simulink model "MIL4L3_SW6_V1_20220211"  (R2018b)
settings: Solver=FixedStepAuto  StartTime=0.0  StopTime=inf  FixedStep=0.001  RelTol=1e-3
PreLoadFcn:
  | A0_MILtest;
undefined symbols (not defined in the file or in its folder): Clb_ICADirect_LaneDisp_StateFive, Clb_ICADirect_LaneDisp_StateFour, Clb_ICADirect_LaneDisp_StateOne, Clb_ICADirect_LaneDisp_StateThree, Clb_ICADirect_LaneDisp_StateTwo, Clb_ICADirect_LaneDisp_StateZero, Clb_ICADirect_LaneDispSW, Clb_ICADirect_TrnLghtsCom_Switch, Clb_ICADirect_TrnLghtsCom_Value, Clb_ICADirect_TrnLghtsCrtl_Inhb, IMAP_Clb_ACU_Driver_Belt, IMAP_Clb_ACU_Driver_Belt_Over, IMAP_Clb_ACU_Passenger_Belt, IMAP_Clb_ACU_Passenger_Belt_Over, IMAP_Clb_ACU_RearLeft_Belt, IMAP_Clb_ACU_RearLeft_Belt_Over, IMAP_Clb_ACU_RearMiddle_Belt, IMAP_Clb_ACU_RearMiddle_Belt_Over, IMAP_Clb_ACU_RearRight_Belt, IMAP_Clb_ACU_RearRight_Belt_Over, IMAP_Clb_AEB_Switch, IMAP_Clb_AEB_Switch_Over, IMAP_Clb_ALC_TLC_Mode, IMAP_Clb_ALC_TLC_Mode_Over, IMAP_Clb_BCM_Battery_Voltage, IMAP_Clb_BCM_Battery_Voltage_Over, IMAP_Clb_BCM_BrakeLamp_State, IMAP_Clb_BCM_BrakeLamp_State_Over, IMAP_Clb_BCM_CHMSL_Status, IMAP_Clb_BCM_CHMSL_Status_Over, IMAP_Clb_BCM_Door_Lock_State, IMAP_Clb_BCM_Door_Lock_State_Over, IMAP_Clb_BCM_FrontWiper_State, IMAP_Clb_BCM_FrontWiper_State_Over, IMAP_Clb_BCM_FrontWiper_Switch, IMAP_Clb_BCM_FrontWiper_Switch_Over, IMAP_Clb_BCM_HazardLamp, IMAP_Clb_BCM_HazardLamp_Over, IMAP_Clb_BCM_HazardLamp_Switch, IMAP_Clb_BCM_HazardLamp_Switch_Over, IMAP_Clb_BCM_HighBeam_State, IMAP_Clb_BCM_HighBeam_State_Over, IMAP_Clb_BCM_Ignition_State, IMAP_Clb_BCM_Ignition_State_Over, IMAP_Clb_BCM_IHBC_Enabled, IMAP_Clb_BCM_IHBC_Enabled_Over, IMAP_Clb_BCM_Left_Light, IMAP_Clb_BCM_Left_Light_Over, IMAP_Clb_BCM_LeftTurn_Switch, IMAP_Clb_BCM_LeftTurn_Switch_Over, IMAP_Clb_BCM_LF_Door_State, IMAP_Clb_BCM_LF_Door_State_Over, IMAP_Clb_BCM_LowBeam_State, IMAP_Clb_BCM_LowBeam_State_Over, IMAP_Clb_BCM_LR_Door_State, IMAP_Clb_BCM_LR_Door_State_Over, IMAP_Clb_BCM_RF_Door_State, IMAP_Clb_BCM_RF_Door_State_Over, IMAP_Clb_BCM_Right_Light, IMAP_Clb_BCM_Right_Light_Over ... (+547)
libraries: CarMaker4SL x2153, simulink x292, dspstat3 x3, canmsglib x2, simulink_extras x1
(part 39 of 52)

== system MIL4L3_SW6_V1_20220211/CarMaker/VehicleControl/Function/LKA/LKAS1/LL/LLOn/LKA Input Processing (LKAInP)/Previewed Heading Angle Calculation (PrHdAg) ==
  PrHdAg_bsInInfoSyn : Inport
  PrHdAg_bsLLClb : Inport  Port=2
  PrHdAg_bsTTLCInfo : Inport  Port=3
  Add1 : Sum  AccumDataTypeStr=single
  Add2 : Sum  AccumDataTypeStr=single
  Bus Creator1 : BusCreator  Inputs=8
  Bus Selector2 : BusSelector  OutputSignals=bsLaneInfo.bsL0Info,bsVehMovInfo.ESC_VehSpd,bsLaneInfo.bsR0Info
  Bus Selector3 : BusSelector  OutputSignals=bsLKAClb.LL_HdAgPrvwT_C
  Bus Selector4 : BusSelector  OutputSignals=LFTTTLC,RGTTTLC
  Compare To Constant : simulink/Logic and Bit Operations/Compare To Constant  relop=<=  const=2  OutDataTypeStr=boolean
  Compare To Constant1 : simulink/Logic and Bit Operations/Compare To Constant  relop=<=  const=2  OutDataTypeStr=boolean
  Gain1 : Gain  Gain=0.5
  Gain2 : Gain  Gain=0.5
  Perdicted Heading Angle from Right Lane Line (PrdcHdAgRgt)1 : Subsystem
  Perdicted Heading Angle from Right Lane Line (PrvwTTLCHdAgLftTTLCRgt) : Subsystem
  Perdicted Heading Angle from Right Lane Line (PrvwTTLCHdAgRgtTTLCRgt) : Subsystem
  Predicted Heading Angle from Left Lane Line (PrdcHdAgtLft)1 : Subsystem
  Predicted Heading Angle from Left Lane Line (PrdcHdAgtLftTTLCLft) : Subsystem
  Predicted Heading Angle from Left Lane Line (PrvwTTLCHdAgRgtTTLCLft) : Subsystem
  Saturation : Saturate  UpperLimit=2  LowerLimit=0.5
      settings: AttributesFormatString="Min = %<LowerLimit>  Max = %<UpperLimit>"
  Saturation1 : Saturate  UpperLimit=2  LowerLimit=0.5
      settings: AttributesFormatString="Min = %<LowerLimit>  Max = %<UpperLimit>"
  Switch : Switch  Criteria=u2 > Threshold
  Switch1 : Switch  Criteria=u2 > Threshold
  Z Calculation (ZCalc) : Subsystem
  Z Calculation (ZCalc)1 : Subsystem
  PrHdAg_bsPrHdAgInfo : Outport
  wires:
  PrHdAg_bsInInfoSyn/1 -> Bus Selector2/1
  Bus Selector2/3 -> Perdicted Heading Angle from Right Lane Line (PrvwTTLCHdAgRgtTTLCRgt)/2(PrdcHdAgRgt_bsR0Info), Perdicted Heading Angle from Right Lane Line (PrdcHdAgRgt)1/2(PrdcHdAgRgt_bsR0Info), Perdicted Heading Angle from Right Lane Line (PrvwTTLCHdAgLftTTLCRgt)/2(PrdcHdAgRgt_bsR0Info)  "<bsR0Info>"
  Z Calculation (ZCalc)/1(ZCalc_lPrvwDstZ) -> Perdicted Heading Angle from Right Lane Line (PrvwTTLCHdAgLftTTLCRgt)/1(PrdcHdAgRgt_lPrvwDstZ), Predicted Heading Angle from Left Lane Line (PrdcHdAgtLftTTLCLft)/2(PrdcHdAgtLft_lPrvwDstZ), Bus Creator1/6, Add1/1  "lPrvwZLft"
  Bus Selector4/1 -> Switch/1, Compare To Constant/1  "<LFTTTLC>"
  Bus Selector2/1 -> Predicted Heading Angle from Left Lane Line (PrvwTTLCHdAgRgtTTLCLft)/1(PrdcHdAgtLft_bsL0Info), Predicted Heading Angle from Left Lane Line (PrdcHdAgtLft)1/1(PrdcHdAgtLft_bsL0Info), Predicted Heading Angle from Left Lane Line (PrdcHdAgtLftTTLCLft)/1(PrdcHdAgtLft_bsL0Info)  "<bsL0Info>"
  Saturation/1 -> Z Calculation (ZCalc)/2(ZCalc_tiHdAgPrvwT_C)
  PrHdAg_bsTTLCInfo/1 -> Bus Selector4/1
  Bus Creator1/1 -> PrHdAg_bsPrHdAgInfo/1
  Bus Selector4/2 -> Switch1/1, Compare To Constant1/1  "<RGTTTLC>"
  Predicted Heading Angle from Left Lane Line (PrdcHdAgtLftTTLCLft)/1(PrdcHdAgtLft_phiPrdcHdAgLft) -> Bus Creator1/1  "phiPrvwTTLCHdAgLftTTLCLft"
  Perdicted Heading Angle from Right Lane Line (PrvwTTLCHdAgRgtTTLCRgt)/1(PrdcHdAgRgt_phiPrdcHdAgRgt) -> Bus Creator1/4  "phiPrvwTTLCHdAgRgtTTLCRgt"
  Bus Selector2/2 -> Z Calculation (ZCalc)1/1(ZCalc_vVehSpd), Z Calculation (ZCalc)/1(ZCalc_vVehSpd)  "<ESC_VehSpd>"
  Add2/1 -> Gain2/1
  Gain2/1 -> Bus Creator1/5  "phiPrvwHdAgMean"
  PrHdAg_bsLLClb/1 -> Bus Selector3/1
  Compare To Constant/1 -> Switch/2
  Switch/1 -> Saturation/1
  Switch1/1 -> Saturation1/1
  Bus Selector3/1 -> Switch/3, Switch1/3  "<LL_HdAgPrvwT_C>"
  Saturation1/1 -> Z Calculation (ZCalc)1/2(ZCalc_tiHdAgPrvwT_C)
  Z Calculation (ZCalc)1/1(ZCalc_lPrvwDstZ) -> Bus Creator1/7, Perdicted Heading Angle from Right Lane Line (PrvwTTLCHdAgRgtTTLCRgt)/1(PrdcHdAgRgt_lPrvwDstZ), Predicted Heading Angle from Left Lane Line (PrvwTTLCHdAgRgtTTLCLft)/2(PrdcHdAgtLft_lPrvwDstZ), Add1/2  "lPrvwZRgt"
  Compare To Constant1/1 -> Switch1/2
  Add1/1 -> Gain1/1
  Gain1/1 -> Predicted Heading Angle from Left Lane Line (PrdcHdAgtLft)1/2(PrdcHdAgtLft_lPrvwDstZ), Perdicted Heading Angle from Right Lane Line (PrdcHdAgRgt)1/1(PrdcHdAgRgt_lPrvwDstZ), Bus Creator1/8  "PrvwZMean"
  Predicted Heading Angle from Left Lane Line (PrdcHdAgtLft)1/1(PrdcHdAgtLft_phiPrdcHdAgLft) -> Add2/1  "phiPrvwTTLCHdAgLft"
  Perdicted Heading Angle from Right Lane Line (PrdcHdAgRgt)1/1(PrdcHdAgRgt_phiPrdcHdAgRgt) -> Add2/2  "phiPrvwTTLCHdAgRgt"
  Predicted Heading Angle from Left Lane Line (PrvwTTLCHdAgRgtTTLCLft)/1(PrdcHdAgtLft_phiPrdcHdAgLft) -> Bus Creator1/2  "phiPrvwTTLCHdAgRgtTTLCLft"
  Perdicted Heading Angle from Right Lane Line (PrvwTTLCHdAgLftTTLCRgt)/1(PrdcHdAgRgt_phiPrdcHdAgRgt) -> Bus Creator1/3  "phiPrvwTTLCHdAgLftTTLCRgt"

== system MIL4L3_SW6_V1_20220211/CarMaker/VehicleControl/Function/LKA/LKAS1/LL/LLOn/LKA Input Processing (LKAInP)/Steering Wheel Position Calculation (SWAPosCal) ==
  SWAPosCal_bsInInfoSyn : Inport
  SWAPosCal_bsLLClb : Inport  Port=2
  Bus Selector : BusSelector  OutputSignals=bsLaneInfo.bsL0Info,bsLaneInfo.bsR0Info,bsVehMovInfo.ESC_VehSpd,bsSWAInfo.SW_Angle
  Bus Selector2 : BusSelector  OutputSignals=bsConstantClb.LKA_SampleTime
  Subsystem : Subsystem
  Subsystem1 : Subsystem
  SWAPosCal : Outport
  wires:
  SWAPosCal_bsInInfoSyn/1 -> Bus Selector/1
  Bus Selector/1 -> Subsystem1/1(L0)  "<bsL0Info>"
  Bus Selector/2 -> Subsystem1/2(R0)  "<bsR0Info>"
  Subsystem1/1(Flg) -> Subsystem/Enable  "SWAPosEna"
  Bus Selector/3 -> Subsystem1/3(VehSpd)  "<ESC_VehSpd>"
  Bus Selector/4 -> Subsystem1/4(SWA), Subsystem/1(SWAIn)  "<SW_Angle>"
  Subsystem/1(SWAPos) -> SWAPosCal/1
  SWAPosCal_bsLLClb/1 -> Bus Selector2/1
  Bus Selector2/1 -> Subsystem1/5(LKA_SampleTime), Subsystem/2(LKA_SampleTime)  "<LKA_SampleTime>"

== system MIL4L3_SW6_V1_20220211/CarMaker/VehicleControl/Function/LKA/LKAS1/LL/LLOn/LKA Input Processing (LKAInP)/TTLC Calculation (TTLCCalc) ==
  bsDvtInfo : Inport
  bsLLClb : Inport  Port=2
  bsInfo : Inport  Port=3
  In4 : Inport  Port=4
  In5 : Inport  Port=5
  Bus Creator : BusCreator  Inputs=4
  Bus Selector1 : BusSelector  OutputSignals=Vy_L0,Vy_R0
  Bus Selector2 : BusSelector  OutputSignals=ILftDvt,IRgtDvt
  Bus Selector3 : BusSelector  OutputSignals=crPrvwCrvtLft,crPrvwCrvtRgt
  Bus Selector4 : BusSelector  OutputSignals=bsLaneInfo.bsL0Info.L0_C0,bsLaneInfo.bsL0Info.L0_C1,bsLaneInfo.bsL0Info.L0_C2,bsLaneInfo.bsR0Info.R0_C0,bsLaneInfo.bsR0Info.R0_C1,bsLaneInfo.bsR0Info.R0_C2,bsVehMovInfo.ESC_VehSpd,bsSWAInfo.SW_Angle
  Bus Selector5 : BusSelector  OutputSignals=bsConstantClb.LKA_WhlBaseL_C,bsConstantClb.LKA_StrRatio_C,bsConstantClb.LKA_Veh2CamW_C
  Constant : Constant  Value=2  OutDataTypeStr=single
  Constant1 : Constant  Value=2  OutDataTypeStr=single
  Degrees to Radians : simulink_extras/Transformations/Degrees to Radians
  Gain2 : Gain  Gain=1/3.6
  MATLAB Function : MATLAB Function  TreatAsAtomicUnit=on
  MATLAB Function1 : MATLAB Function  TreatAsAtomicUnit=on
  MATLAB Function2 : MATLAB Function  TreatAsAtomicUnit=on
  MATLAB Function3 : MATLAB Function  TreatAsAtomicUnit=on
  MATLAB Function4 : MATLAB Function  TreatAsAtomicUnit=on
  MATLAB Function5 : MATLAB Function  TreatAsAtomicUnit=on
  Saturation : Saturate  UpperLimit=2  LowerLimit=0.6  OutDataTypeStr=single
      settings: AttributesFormatString="Min = %<LowerLimit>  Max = %<UpperLimit>"
  Saturation1 : Saturate  UpperLimit=2  LowerLimit=0.6  OutDataTypeStr=single
      settings: AttributesFormatString="Min = %<LowerLimit>  Max = %<UpperLimit>"
  Saturation2 : Saturate  UpperLimit=2  LowerLimit=-2
      settings: AttributesFormatString="Min = %<LowerLimit>  Max = %<UpperLimit>"
  Saturation3 : Saturate  UpperLimit=2  LowerLimit=-2
      settings: AttributesFormatString="Min = %<LowerLimit>  Max = %<UpperLimit>"
  Saturation7 : Saturate  UpperLimit=2  LowerLimit=0.8
      settings: AttributesFormatString="Min = %<LowerLimit>  Max = %<UpperLimit>"
  Saturation8 : Saturate  UpperLimit=2  LowerLimit=0.8
      settings: AttributesFormatString="Min = %<LowerLimit>  Max = %<UpperLimit>"
  Unary Minus1 : UnaryMinus
  TTLCCalc_bsTTLCInfo : Outport
  tag scope: LFTTTLC_Mon=global, RGTTTLC_Mon=global
  wires:
  Saturation3/1 -> [VxR0]
  Saturation2/1 -> [VxL0]
  Unary Minus1/1 -> Saturation2/1
  Bus Selector1/2 -> Saturation3/1  "<Vy_R0>"
  Bus Selector1/1 -> Unary Minus1/1  "<Vy_L0>"
  In5/1 -> Bus Selector1/1
  In4/1 -> Bus Selector3/1
  Bus Selector3/1 -> [CurL]  "<crPrvwCrvtLft>"
  Bus Selector3/2 -> [CurR]  "<crPrvwCrvtRgt>"
  Gain2/1 -> MATLAB Function5/1(vx), [Vx]
  Bus Selector4/7 -> Gain2/1  "<ESC_VehSpd>"
  bsLLClb/1 -> Bus Selector5/1
  bsInfo/1 -> Bus Selector4/1
  bsDvtInfo/1 -> Bus Selector2/1
  Bus Selector2/2 -> MATLAB Function1/1(dvt)  "<IRgtDvt>"
  [VxL0] -> MATLAB Function/2(vy)
  [VxR0] -> MATLAB Function1/2(vy)
  MATLAB Function1/1(TTLC) -> Saturation1/1  "RGTLC"
  MATLAB Function/1(TTLC) -> Saturation/1
  Saturation/1 -> [LftTTLC]  "LftTTLC"
  Saturation1/1 -> [RgtTTLC]  "RgtTTLC"
  Bus Selector2/1 -> MATLAB Function/1(dvt)  "<ILftDvt>"
  [CurR] -> MATLAB Function1/3(cur)
  [CurL] -> MATLAB Function/3(cur)
  Bus Selector4/5 -> [R0C1]  "<R0_C1>"
  Bus Selector4/4 -> [R0C0]  "<R0_C0>"
  Bus Selector4/6 -> [R0C2]  "<R0_C2>"
  Bus Selector4/2 -> [L0C1]  "<L0_C1>"
  Bus Selector4/1 -> [L0C0]  "<L0_C0>"
  Bus Selector4/3 -> [L0C2]  "<L0_C2>"
  [C20] -> MATLAB Function3/5(c20)
  MATLAB Function4/1(TRgt) -> [TRgt]  "TRgt"
  [R0C2] -> MATLAB Function4/3(c2)
  [Vx] -> MATLAB Function3/4(vx)
  [C20] -> MATLAB Function4/5(c20)
  [W] -> MATLAB Function4/6(w)
  [R0C0] -> MATLAB Function4/1(c0)
  MATLAB Function3/1(TLft) -> [TLft]  "TLft"
  [L0C1] -> MATLAB Function3/2(c1)
  [W] -> MATLAB Function3/6(w)
  [R0C1] -> MATLAB Function4/2(c1)
  [Vx] -> MATLAB Function4/4(vx)
  [L0C2] -> MATLAB Function3/3(c2)
  [L0C0] -> MATLAB Function3/1(c0)
  Bus Creator/1 -> TTLCCalc_bsTTLCInfo/1
  [TLft] -> MATLAB Function2/7(TLft)
  [LftTTLC] -> MATLAB Function2/5(LTTLC)
  [TRgt] -> MATLAB Function2/8(TRgt)
  Saturation7/1 -> [LFTTTLC_Mon], Bus Creator/1  "LFTTTLC"
  [CurL] -> MATLAB Function2/1(crPrvwCrvtLft)
  MATLAB Function2/1(LFTTTLC) -> Saturation7/1  "LFTTTLC"
  [RgtTTLC] -> MATLAB Function2/6(RTTLC)
  MATLAB Function2/2(RGTTTLC) -> Saturation8/1  "RGTTTLC"
  Saturation8/1 -> Bus Creator/2, [RGTTTLC_Mon]  "RGTTTLC"
  [CurR] -> MATLAB Function2/2(crPrvwCrvtRgt)
  Bus Selector4/8 -> Degrees to Radians/1  "<SW_Angle>"
  Degrees to Radians/1 -> MATLAB Function5/2(sw_angle)
  Bus Selector5/1 -> MATLAB Function5/3(WhlBaseL_C)  "<LKA_WhlBaseL_C>"
  MATLAB Function5/1(TTLC) -> [C20]
  Bus Selector5/3 -> [W]  "<LKA_Veh2CamW_C>"
  Bus Selector5/2 -> MATLAB Function5/4(StrRatio_C)  "<LKA_StrRatio_C>"
  [VxL0] -> Bus Creator/3  "vLft"
  [VxR0] -> Bus Creator/4  "vRgt"
  [LTLC] -> MATLAB Function2/3(LTLC)
  [RTLC] -> MATLAB Function2/4(RTLC)
  Constant/1 -> [LTLC]
  Constant1/1 -> [RTLC]

== system MIL4L3_SW6_V1_20220211/CarMaker/VehicleControl/Function/LKA/LKAS1/LL/LLOn/LKA Input Processing (LKAInP)/Under The Limit (UndrLim) ==
  UndrLim_bsInInfoSyn : Inport
  UndrLim_bsLLClb : Inport  Port=2
  Bus Creator : BusCreator  Inputs=2
  Bus Selector1 : BusSelector  OutputSignals=bsVehMovInfo.ESC_VehSpd
  Bus Selector2 : BusSelector  OutputSignals=bsLKAClb.LL_LAccMax_C,bsLKAClb.LL_LAccRMax_C,bsConstantClb.LKA_StrRatio_C,bsConstantClb.LKA_WhlBaseL_C
  Saturation : Saturate  UpperLimit=150  LowerLimit=0.001
      settings: AttributesFormatString="Min = %<LowerLimit>  Max = %<UpperLimit>"
  Steering Wheel Angel Max (SWAMax) : Subsystem
  Steering Wheel Angel Rate Max (SWARMax) : Subsystem
  UndrLim_bsUndrLimInfo : Outport
  wires:
  Saturation/1 -> Steering Wheel Angel Rate Max (SWARMax)/1(SWARateMax_vVehSpd), Steering Wheel Angel Max (SWAMax)/1(SWAMax_vVehSpd)
  Steering Wheel Angel Rate Max (SWARMax)/1(SWARMax_dphiSWARMax) -> Bus Creator/2  "UndrLim_dphiSWARMax"
  Steering Wheel Angel Max (SWAMax)/1(SWAMax_phiSWAMax) -> Bus Creator/1  "UndrLim_phiSWAMax"
  UndrLim_bsInInfoSyn/1 -> Bus Selector1/1
  Bus Selector1/1 -> Saturation/1  "<ESC_VehSpd>"
  UndrLim_bsLLClb/1 -> Bus Selector2/1
  Bus Selector2/1 -> Steering Wheel Angel Max (SWAMax)/2(SWAMax_aLAcc_C)  "<LL_LAccMax_C>"
  Bus Selector2/2 -> Steering Wheel Angel Rate Max (SWARMax)/2(SWARateMax_aLAccR_C)  "<LL_LAccRMax_C>"
  Bus Selector2/3 -> Steering Wheel Angel Rate Max (SWARMax)/3(LKA_StrRatio_C), Steering Wheel Angel Max (SWAMax)/3(LKA_StrRatio_C)  "<LKA_StrRatio_C>"
  Bus Selector2/4 -> Steering Wheel Angel Max (SWAMax)/4(LKA_WhlBaseL_C), Steering Wheel Angel Rate Max (SWARMax)/4(LKA_WhlBaseL_C)  "<LKA_WhlBaseL_C>"
  Bus Creator/1 -> UndrLim_bsUndrLimInfo/1

== system MIL4L3_SW6_V1_20220211/CarMaker/VehicleControl/Function/LKA/LKAS1/LL/LLOn/LL State Determination (LLStateDet)/LL State Machine Conditions (LLSMCon) ==
  LLSMCon_bsInInfoSyn : Inport
  LLSMCon_bsLKAInPInfo : Inport  Port=2
  LLSMCon_bsLLClb : Inport  Port=3
  LLSMCon_bsLLState : Inport  Port=4
  LLSMCon_stExitFlg : Inport  Port=5
  LLSMCon_bsSignalFault : Inport  Port=6
  Activation Condition (ActvC) : Subsystem  Description=|
      | Block Name: Activation Condition
      | Ab.: ActvC
      | No.: 1.1.1.4.0.
      | Rev: 0.0.1
      | Update Date: 19-3-26
  Bus Selector : BusSelector  OutputSignals=bsMP5Info.LKA_Mode
  Cast : DataTypeConversion
  Cast1 : DataTypeConversion
  Deactivation Condition (DeactvC) : Subsystem  Description=|
      | Block Name: Deactivation Condition
      | Ab.: DeactvC
      | No.: 1.1.1.5.0.0
      | Rev: 0.0.1
      | Update Date: 19-3-26
  Disable Condition (DisblC) : Subsystem  Description=|
      | Block Name: Disable Condition
      | Ab.: DisblC
      | No.: 1.1.1.3.0.0
      | Rev: 0.0.1
      | Update Date: 19-3-26
  Enable Condition (EnaC) : Subsystem  Description=|
      | Block Name: Enable Condition
      | Ab.: EnaC
      | No.: 1.1.1.2.0.0
      | Rev: 0.0.1
      | Update Date: 19-3-26
      settings: PermitHierarchicalResolution=None  MinAlgLoopOccurrences=on
  Fault Condition (FaultC) : Subsystem  Description=|
      | Block Name: Fault Condition
      | Ab.: FaultC
      | No.: 1.1.1.6.0.0
      | Rev: 0.0.1
      | Update Date: 19-3-26
  Terminator : Terminator
  Terminator1 : Terminator
  LLSMCon_stDACMode : Outport
  LLSMCon_stLDWEnaCSyn : Outport  Port=2
  LLSMCon_stLDWDisblCSyn : Outport  Port=3
  LLSMCon_stLDWActvCSyn : Outport  Port=4
  LLSMCon_stLDWDeactvCSyn : Outport  Port=5
  LLSMCon_stLDWFaultCSyn : Outport  Port=6
  LLSMCon_stLKAEnaCSyn : Outport  Port=7
  LLSMCon_stLKADisblCSyn : Outport  Port=8
  LLSMCon_stLKAActvCSyn : Outport  Port=9
  LLSMCon_stLKADeactvCSyn : Outport  Port=10
  LLSMCon_stLKAFaultCSyn : Outport  Port=11
  Disable_Reason : Outport  Port=12
  wires:
  Enable Condition (EnaC)/2(EnaC_stLKAEnaCSyn) -> LLSMCon_stLKAEnaCSyn/1
  Disable Condition (DisblC)/1(DisblC_stLDWDisblCSyn) -> LLSMCon_stLDWDisblCSyn/1
  Disable Condition (DisblC)/2(DisblC_stLKADisblCSyn) -> LLSMCon_stLKADisblCSyn/1
  Enable Condition (EnaC)/1(EnaC_stLDWEnaCSyn) -> LLSMCon_stLDWEnaCSyn/1
  LLSMCon_bsLLState/1 -> Deactivation Condition (DeactvC)/5(LLState), Disable Condition (DisblC)/5(LLState)
  LLSMCon_bsInInfoSyn/1 -> Bus Selector/1, Enable Condition (EnaC)/2(EnaC_bsInInfoSyn), Fault Condition (FaultC)/1(FaultC_bsInInfoSyn), Deactivation Condition (DeactvC)/2(InInfoSyn), Activation Condition (ActvC)/2(InInfoSyn), Disable Condition (DisblC)/2(InInfoSyn)
  Activation Condition (ActvC)/1(ActvC_stLDWActvCSyn) -> LLSMCon_stLDWActvCSyn/1
  Fault Condition (FaultC)/1(FaultC_stLDWFaultCSyn) -> LLSMCon_stLDWFaultCSyn/1
  Deactivation Condition (DeactvC)/2(DeactvC_stLKADeactvCSyn) -> LLSMCon_stLKADeactvCSyn/1, Cast1/1
  Fault Condition (FaultC)/2(FaultC_stLKAFaultCSyn) -> LLSMCon_stLKAFaultCSyn/1
  Deactivation Condition (DeactvC)/1(DeactvC_stLDWDeactvCSyn) -> LLSMCon_stLDWDeactvCSyn/1
  LLSMCon_stExitFlg/1 -> Deactivation Condition (DeactvC)/6(ExitFlg)
  LLSMCon_bsLLClb/1 -> Fault Condition (FaultC)/2(FaultC_bsLLClb), Deactivation Condition (DeactvC)/4(LLClb), Activation Condition (ActvC)/4(LLClb), Disable Condition (DisblC)/4(LLClb), Enable Condition (EnaC)/4(EnaC_bsLLClb)
  Activation Condition (ActvC)/2(ActvC_stLKAActvCSyn) -> LLSMCon_stLKAActvCSyn/1
  LLSMCon_bsSignalFault/1 -> Fault Condition (FaultC)/3(FaultC_SignalFault)
  LLSMCon_bsLKAInPInfo/1 -> Deactivation Condition (DeactvC)/3(LKAInPInfo), Activation Condition (ActvC)/3(LKAInPInfo), Disable Condition (DisblC)/3(LKAInPInfo), Enable Condition (EnaC)/3(EnaC_bsLKAInPInfo)
  Bus Selector/1 -> Deactivation Condition (DeactvC)/1(DACMode), Activation Condition (ActvC)/1(DACMode), Disable Condition (DisblC)/1(DACMode), Enable Condition (EnaC)/1(EnaC_stDACMode), LLSMCon_stDACMode/1  "<LKA_Mode>"
  Cast/1 -> Terminator/1  "ob_LKA_Disable_Reason"
  Disable Condition (DisblC)/3(Disable_Reason) -> Disable_Reason/1, Cast/1  "Disable_Reason"
  Cast1/1 -> Terminator1/1  "ob_LKA_LKADeactvCSyn"

== system MIL4L3_SW6_V1_20220211/CarMaker/VehicleControl/Function/LKA/LKAS1/LL/LLOut/Angle2Trq/Rate Limiter Dynamic ==
  note: U(k)
  note: Y(k)
  up : Inport
  u : Inport  Port=2
  lo : Inport  Port=3
  Delay Input2 : UnitDelay  Description=Store in Global RAM  DisableCoverage=on  SampleTime=-1
  Difference Inputs1 : Sum  Description=Add in CPU  DisableCoverage=on  Inputs=+-  OutDataTypeStr=Inherit: Inherit via back propagation
  Difference Inputs2 : Sum  Description=Add in CPU  OutDataTypeStr=Inherit: Inherit via back propagation
  FixPt Data Type Duplicate : DataTypeDuplicate  DisableCoverage=on  NumInputPorts=7
  Saturation Dynamic : simulink/Discontinuities/Saturation Dynamic  OutMin=[]  OutMax=[]  OutDataTypeStr=Inherit: Same as second input  OutDataType=fixdt(1, 16)  OutScaling=2^-10  DoSatur=off
  delta fall limit : Product  DisableCoverage=on  Inputs=**  OutDataTypeStr=Inherit: Inherit via back propagation  SaturateOnIntegerOverflow=on
  delta rise limit : Product  DisableCoverage=on  Inputs=**  OutDataTypeStr=Inherit: Inherit via back propagation  SaturateOnIntegerOverflow=on
  sample time : SampleTimeMath  DisableCoverage=on  TsampMathOp=Ts Only  weightValue=1
  Y : Outport  InitialOutput=0
  wires:
  u/1 -> sample time/1, FixPt Data Type Duplicate/5, Difference Inputs1/1
  delta fall limit/1 -> Saturation Dynamic/3, FixPt Data Type Duplicate/3
  up/1 -> delta rise limit/1
  sample time/1 -> delta rise limit/2, delta fall limit/2
  Saturation Dynamic/1 -> FixPt Data Type Duplicate/7, Difference Inputs2/1
  delta rise limit/1 -> Saturation Dynamic/1, FixPt Data Type Duplicate/6
  Difference Inputs1/1 -> Saturation Dynamic/2, FixPt Data Type Duplicate/4  "( U(k) - Y(k-1) )"
  lo/1 -> delta fall limit/1
  Delay Input2/1 -> Difference Inputs2/2, FixPt Data Type Duplicate/2, Difference Inputs1/2  "Y(k-1)"
  Difference Inputs2/1 -> FixPt Data Type Duplicate/1, Delay Input2/1, Y/1

== system MIL4L3_SW6_V1_20220211/CarMaker/VehicleControl/Function/LKA/LKAS1/LL/LLOut/Angle2Trq/Saturation Dynamic ==
  up : Inport
  u : Inport  Port=2
  lo : Inport  Port=3
  Data Type Duplicate : DataTypeDuplicate  DisableCoverage=on
  Data Type Propagation : simulink/Signal Attributes/Data Type Propagation  PropDataType=fixdt(1, 16)  IfRefDouble=double  IfRefSingle=single  IsSigned=IsSigned1  NumBitsBase=NumBits1  NumBitsMult=1  NumBitsAdd=0  NumBitsAllowFinal=1:128  PropScaling=2^-10  ValuesUsedBestPrec=[5 -7]  SlopeBase=Slope1  SlopeMult=1  SlopeAdd=0  BiasBase=Bias1  BiasMult=1  BiasAdd=0
      settings: SourceProductName=Simulink  SourceProductBaseCode=SL
  LowerRelop1 : RelationalOperator  DisableCoverage=on  Operator=>  OutDataTypeStr=boolean  RndMeth=Nearest
  Switch : Switch  Criteria=u2 ~= 0  OutDataTypeStr=Inherit: Inherit via back propagation  ZeroCross=off
  Switch2 : Switch  Criteria=u2 ~= 0  OutDataTypeStr=Inherit: Inherit via back propagation  ZeroCross=off
  UpperRelop : RelationalOperator  DisableCoverage=on  Operator=<  OutDataTypeStr=boolean  RndMeth=Nearest
  y : Outport
  wires:
  LowerRelop1/1 -> Switch2/2
  Switch2/1 -> Data Type Duplicate/1, y/1
  lo/1 -> UpperRelop/2, Switch/1
  up/1 -> LowerRelop1/2, Switch2/1
  u/1 -> UpperRelop/1, Switch/3, LowerRelop1/1, Data Type Propagation/1, Data Type Propagation/2
  UpperRelop/1 -> Switch/2
  Switch/1 -> Data Type Propagation/3, Switch2/3, Data Type Duplicate/2

== system MIL4L3_SW6_V1_20220211/CarMaker/VehicleControl/Function/LKA/LKAS1/LL/LLOut/Angle2Trq/Subsystem ==
  Target_Angle : Inport
  Stearing_Angle : Inport  Port=2
  Enable : EnablePort  StatesWhenEnabling=reset
  Add : Sum  Inputs=+-
  Add1 : Sum
  Add2 : Sum  Inputs=+++
  Delay1 : Delay  DelayLength=1
  Fcn : Fcn  Expr=u(1)*u(1)*u(1)*0.000002+u(1)*u(1)*(-0.0005)+u(1)*0.0505
  Ki : Constant  Value=0.0005  OutDataTypeStr=single
  Kp : Constant  Value=0.02  OutDataTypeStr=single
  Product1 : Product
  Product2 : Product
  Saturation : Saturate
  in_trq : Outport  OutputWhenDisabled=reset  InitialOutput=0
  wires:
  Add1/1 -> Saturation/1
  Target_Angle/1 -> Add/1, Fcn/1
  Product1/1 -> Add2/2  "Kp"
  Kp/1 -> Product1/2
  Delay1/1 -> Add1/2
  Saturation/1 -> Delay1/1, Add2/3  "Ki"
  Product2/1 -> Add1/1
  Add/1 -> Product2/1, Product1/1  "derta_angle"
  Ki/1 -> Product2/2
  Fcn/1 -> Add2/1  "Kf"
  Add2/1 -> in_trq/1  "in_trq"
  Stearing_Angle/1 -> Add/2

== system MIL4L3_SW6_V1_20220211/CarMaker/VehicleControl/OMAP/OMAP1/Runnable_OMAP_10ms_sys/OMAP_Module/ACCS_Direct/ACCS_Define/ACC_State_Synthesis(ACC_SS) ==
  Input_ACCS : Inport
  Bus Selector : BusSelector  OutputSignals=Deceleration_setpoint_device,TminDownGear,TminUpGear,StAcvTqWhlPTPotReq,PotACCTqReq,Function_Acc_status,ACCTqReq,Powertrain_torquewheel_request,TYPE_RAPPORT,MDD_Decelerationcontrol_request,MDD_deceleration_type,Power_steering_power_cut3F2
  Bus Selector2 : BusSelector  OutputSignals=ACCSve_d_ACC_State_convert
  Compare To Constant1 : simulink/Logic and Bit Operations/Compare To Constant  relop===  const=0  OutDataTypeStr=boolean
  Compare To Constant2 : simulink/Logic and Bit Operations/Compare To Constant  relop===  const=1  OutDataTypeStr=boolean
  Compare To Constant5 : simulink/Logic and Bit Operations/Compare To Constant  relop===  const=2  OutDataTypeStr=boolean
  Compare To Constant6 : simulink/Logic and Bit Operations/Compare To Constant  relop===  const=3  OutDataTypeStr=boolean
  Compare To Constant7 : simulink/Logic and Bit Operations/Compare To Constant  relop===  const=15  OutDataTypeStr=boolean
  If Action Subsystem2 : Subsystem  TreatAsAtomicUnit=on
  If Action Subsystem3 : Subsystem  TreatAsAtomicUnit=on
  If1 : If  IfExpression=u1 == 1
  Logical Operator1 : Logic  Operator=OR  Inputs=5  AllPortsSameDT=off  OutDataTypeStr=boolean
  Merge : Merge
  ACC_Control_Signal : Outport
  tag scope: ob_ACC_ACCTqReq=global, ob_ACC_Deceleration_setpoint_device=global, ob_ACC_Function_Acc_status=global, ob_ACC_MDD_Decelerationcontrol_request=global, ob_ACC_MDD_deceleration_type=global, ob_ACC_PotACCTqReq=global, ob_ACC_Power_steering_power_cut3F2=global, ob_ACC_Powertrain_torquewheel_request=global, ob_ACC_StAcvTqWhlPTPotReq=global, ob_ACC_TYPE_RAPPORT=global, ob_ACC_TminDownGear=global, ob_ACC_TminUpGear=global
  wires:
  Input_ACCS/1 -> Bus Selector2/1, If Action Subsystem3/1(ACT_Control_Signal)
  Bus Selector/12 -> [ob_ACC_Power_steering_power_cut3F2]  "<Power_steering_power_cut3F2>"
  Bus Selector/11 -> [ob_ACC_MDD_deceleration_type]  "<MDD_deceleration_type>"
  Bus Selector/10 -> [ob_ACC_MDD_Decelerationcontrol_request]  "<MDD_Decelerationcontrol_request>"
  Bus Selector/9 -> [ob_ACC_TYPE_RAPPORT]  "<TYPE_RAPPORT>"
  Bus Selector/8 -> [ob_ACC_Powertrain_torquewheel_request]  "<Powertrain_torquewheel_request>"
  Bus Selector/7 -> [ob_ACC_ACCTqReq]  "<ACCTqReq>"
  Bus Selector/6 -> [ob_ACC_Function_Acc_status]  "<Function_Acc_status>"
  Bus Selector/5 -> [ob_ACC_PotACCTqReq]  "<PotACCTqReq>"
  Bus Selector/4 -> [ob_ACC_StAcvTqWhlPTPotReq]  "<StAcvTqWhlPTPotReq>"
  Bus Selector/3 -> [ob_ACC_TminUpGear]  "<TminUpGear>"
  Bus Selector/2 -> [ob_ACC_TminDownGear]  "<TminDownGear>"
  Bus Selector/1 -> [ob_ACC_Deceleration_setpoint_device]  "<Deceleration_setpoint_device>"
  Merge/1 -> ACC_Control_Signal/1, Bus Selector/1  "Control_Ouput"
  If Action Subsystem3/1(Control_Ouput) -> Merge/2
  If Action Subsystem2/1(Control_Ouput) -> Merge/1
  If1/2 -> If Action Subsystem3/Action
  If1/1 -> If Action Subsystem2/Action
  Logical Operator1/1 -> If1/1
  Compare To Constant7/1 -> Logical Operator1/5
  Compare To Constant6/1 -> Logical Operator1/4
  Compare To Constant5/1 -> Logical Operator1/3
  Compare To Constant1/1 -> Logical Operator1/1
  Compare To Constant2/1 -> Logical Operator1/2
  Bus Selector2/1 -> Compare To Constant1/1, Compare To Constant2/1, Compare To Constant5/1, Compare To Constant6/1, Compare To Constant7/1, If Action Subsystem2/1(In1)  "<ACCSve_d_ACC_State_convert>"

== system MIL4L3_SW6_V1_20220211/CarMaker/VehicleControl/OMAP/OMAP1/Runnable_OMAP_10ms_sys/OMAP_Module/ACCS_Direct/ACCS_Define/Human_Machine_Interface(ACC_HMI) ==
  CIPV_ID_Longitudinal_Distance : Inport
  CIPV_ID : Inport  Port=2
  ACC_State : Inport  Port=3
  ACCActive_Signal : Inport  Port=4
  ACC_ICA_Flag : Inport  Port=5
  HeadWaySet : Inport  Port=6
  VelocitySet : Inport  Port=7
  ACC_go_request : Inport  Port=8
  ACC_DecReq : Inport  Port=9
  Bus Selector : BusSelector  OutputSignals=ACC_Vehicle_Icon_Display,ACC_Set_Speed_Display,ACC_DesiredHeadway_Icon_Basic,RVVACC_Vehiclespeed_request_type
  Gain : Gain  OutDataTypeStr=uint8
  Gain1 : Gain  OutDataTypeStr=uint8
  Subsystem : Subsystem
  Subsystem9 : Subsystem
  Text_PopUp : Subsystem
  ACC_DesiredHeadway_Display : Outport
  ACC_DesiredHeadway_Icon_Basic : Outport  Port=2
  ACC_Desired_Set_Speed : Outport  Port=3
  ACC_Set_Speed_Display : Outport  Port=4
  ACC_Vehicle_Icon_Display : Outport  Port=5
  RVVACC_Vehiclespeed_request_type : Outport  Port=6
  ACC_Pop_Up_Message : Outport  Port=7
  ACC_HMI_TgDisp_Flag : Outport  Port=8
  TARGET_POSITION : Outport  Port=9
  ACC_Pop_Up_Message_TJA : Outport  Port=10
  wires:
  VelocitySet/1 -> Gain/1, Subsystem9/3(VelocitySet)
  HeadWaySet/1 -> Gain1/1
  Subsystem9/1(Out1) -> Bus Selector/1
  Gain/1 -> ACC_Desired_Set_Speed/1  "ACC_Desired_Set_Speed"
  CIPV_ID_Longitudinal_Distance/1 -> Subsystem/1(Distance)
  Subsystem/2(TgDisp_Flag) -> ACC_HMI_TgDisp_Flag/1  "ACC_HMI_TgDisp_Flag"
  Subsystem/1(TARGET_POSITION) -> TARGET_POSITION/1  "TARGET_POSITION"
  CIPV_ID/1 -> Subsystem/2(CIPV_ID)
  Gain1/1 -> ACC_DesiredHeadway_Display/1  "ACC_DesiredHeadway_Display"
  Text_PopUp/1(For4F7) -> ACC_Pop_Up_Message/1  "ACC_Pop_Up_Message"
  Bus Selector/1 -> ACC_Vehicle_Icon_Display/1  "<ACC_Vehicle_Icon_Display>"
  Bus Selector/3 -> ACC_DesiredHeadway_Icon_Basic/1  "<ACC_DesiredHeadway_Icon_Basic>"
  Bus Selector/4 -> RVVACC_Vehiclespeed_request_type/1  "<RVVACC_Vehiclespeed_request_type>"
  Bus Selector/2 -> ACC_Set_Speed_Display/1  "<ACC_Set_Speed_Display>"
  ACCActive_Signal/1 -> Text_PopUp/3(ACCActive_Signal)
  Text_PopUp/2(ForTJA) -> ACC_Pop_Up_Message_TJA/1  "ACC_Pop_Up_Message_TJA"
  ACC_go_request/1 -> Text_PopUp/4(go_request)
  ACC_State/1 -> Subsystem9/1(ACC_State), Text_PopUp/1(ACC_State), Subsystem/3(ACC_State)
  ACC_ICA_Flag/1 -> Subsystem9/2(ACCICA_Flag), Text_PopUp/2(ACCICA_Flag)
  ACC_DecReq/1 -> Text_PopUp/5(ACC_DecReq)

== system MIL4L3_SW6_V1_20220211/CarMaker/VehicleControl/OMAP/OMAP1/Runnable_OMAP_10ms_sys/OMAP_Module/ICA_Direct_G59/ICA_Define/ICA_EPS ==
  EPSPCEM_stICAState : Inport
  angle : Inport  Port=2
  torque_Req : Inport  Port=3
  torque : Inport  Port=4
  EPSPCEM_stEPSCtlState : Inport  Port=5
  Data Type Conversion : DataTypeConversion  OutDataTypeStr=uint16
  Data Type Conversion1 : DataTypeConversion  OutDataTypeStr=single
  Data Type Conversion2 : DataTypeConversion  OutDataTypeStr=uint16
  Data Type Conversion3 : DataTypeConversion  OutDataTypeStr=single
  Data Type Conversion4 : DataTypeConversion  OutDataTypeStr=single
  EPS_Ctr_Disable : Subsystem  TreatAsAtomicUnit=on
  EPS_Ctr_Enable : Subsystem  TreatAsAtomicUnit=on
  If1 : If  IfExpression=u1==3
  Merge{1..5} (5 alike) : Merge
  stEPS_State_Ctl_CMD : Outport
  LKA_TRQ_FACT_REQ : Outport  Port=2
  LKA_OR_LPA_REQ : Outport  Port=3
  ICA_STATE : Outport  Port=4
  ICABve_g_SteerAngleCmd_convert : Outport  Port=5
  ICABve_d_LKATorqueReq_convert : Outport  Port=6
  ICABve_g_LKATorqueReq_Value_convert : Outport  Port=7
  wires:
  Merge1/1 -> Data Type Conversion/1
  EPSPCEM_stEPSCtlState/1 -> EPS_Ctr_Disable/1(stEPSCtlState), EPS_Ctr_Enable/1(stEPSCtlState)
  EPS_Ctr_Enable/1(stEPSCtlCMD) -> Merge1/1
  If1/2 -> EPS_Ctr_Disable/Action
  EPS_Ctr_Enable/2(LKA_TRQ_FACT_REQ) -> Merge2/1
  EPS_Ctr_Disable/2(LKA_TRQ_FACT_REQ) -> Merge2/2
  Merge2/1 -> Data Type Conversion1/1
  EPSPCEM_stICAState/1 -> ICA_STATE/1, If1/1
  Data Type Conversion1/1 -> LKA_TRQ_FACT_REQ/1  "LKA_TRQ_FACT_REQ"
  EPS_Ctr_Disable/1(stEPSCtlCMD) -> Merge1/2
  If1/1 -> EPS_Ctr_Enable/Action
  Data Type Conversion/1 -> stEPS_State_Ctl_CMD/1
  EPS_Ctr_Enable/3(LKA_OR_LPA_REQ) -> Merge3/1
  Data Type Conversion2/1 -> LKA_OR_LPA_REQ/1
  Merge3/1 -> Data Type Conversion2/1
  EPS_Ctr_Disable/3(LKA_OR_LPA_REQ) -> Merge3/2
  Data Type Conversion3/1 -> ICABve_g_SteerAngleCmd_convert/1
  Merge5/1 -> Data Type Conversion4/1
  Merge4/1 -> Data Type Conversion3/1
  Data Type Conversion4/1 -> ICABve_g_LKATorqueReq_Value_convert/1
  EPS_Ctr_Disable/5(torque1) -> Merge5/2
  EPS_Ctr_Disable/4(angle1) -> Merge4/2
  angle/1 -> EPS_Ctr_Enable/2(angle)
  torque/1 -> EPS_Ctr_Enable/3(torque)
  EPS_Ctr_Enable/4(angle1) -> Merge4/1
  EPS_Ctr_Enable/5(torque1) -> Merge5/1
  torque_Req/1 -> ICABve_d_LKATorqueReq_convert/1

== system MIL4L3_SW6_V1_20220211/CarMaker/VehicleControl/OMAP/OMAP1/Runnable_OMAP_10ms_sys/OMAP_Module/ICA_Direct_G59/ICA_Define/Subsystem1 ==
  note: 是否禁止控转向灯标定量
      | 1：禁止
      | 0：不禁止
  note: 0：Default value
      | 1：Left indicator ON
      | 2：Right indicator ON
      | 3：Reserved
  note: 输出转向灯控制指令信号
  note: 0 属于CD状态不输出任何Req
      | 1 属于Start状态开始Judge输出L or R
      | 2 Left推荐变道使能
      | 3 Right 推荐变道使能
  VehMovRx_VehicleStationary : Inport
  L0C0_Org : Inport  Port=2
  L0C1_Org : Inport  Port=3
  L0C2_Org : Inport  Port=4
  L0C3_Org : Inport  Port=5
  R0C0_Org : Inport  Port=6
  R0C1_Org : Inport  Port=7
  R0C2_Org : Inport  Port=8
  R0C3_Org : Inport  Port=9
  ACC_State : Inport  Port=10
  ACC_HMI_Txt_Disp : Inport  Port=11
  EPSRx_stHandOff : Inport  Port=12
  EPSRx_stTkOvStChk : Inport  Port=13
  L0QI_Opt : Inport  Port=14
  R0QI_Opt : Inport  Port=15
  stTHState : Inport  Port=16
  stTHFKeyStt : Inport  Port=17
  stSWALimFlg : Inport  Port=18
  stTHMode : Inport  Port=19
  stLCScene : Inport  Port=20
  stLCmode : Inport  Port=21
  stLCfailedFlg : Inport  Port=22
  HMI_tfAddVocCmd : Inport  Port=23
  stLCRMode : Inport  Port=24
  stLCRmode_valid : Inport  Port=25
  stturn_lightState : Inport  Port=26
  stTLC_ALCmodeSW : Inport  Port=27
  stLC_SpdCndtFlg : Inport  Port=28
  HMI_Clb : Inport  Port=29
  Bus Creator : BusCreator  Inputs=2
  Bus Selector1 : BusSelector  OutputSignals=TH_HMIClb_tiDgrdIconWarnHiDurT_C,TH_HMIClb_tiDgrdIconWarnLoDurT_C,ISA_Value,ISA_TYPE,Mode_tmp,LCScene_tmp
  Compare To Constant : simulink/Logic and Bit Operations/Compare To Constant  relop===  const=4  OutDataTypeStr=boolean
  Compare To Zero1 : simulink/Logic and Bit Operations/Compare To Zero  relop===  OutDataTypeStr=boolean
  Compare To Zero2 : simulink/Logic and Bit Operations/Compare To Zero  relop===  OutDataTypeStr=boolean
  Constant : Constant  Value=0  OutDataTypeStr=uint16
  Constant1 : Constant  Value=0  OutDataTypeStr=uint16
  Constant2 : Constant  Value=0  OutDataTypeStr=uint16
  Constant3 : Constant  Value=Clb_ICADirect_TrnLghtsCrtl_Inhb  OutDataTypeStr=uint16
  Count1 : MATLAB Function  TreatAsAtomicUnit=on
  Data Type Conversion{,3..7,14..17,22,24,35..40,45} (19 alike) : DataTypeConversion  OutDataTypeStr=uint16
  Data Type Conversion1 : DataTypeConversion  OutDataTypeStr=uint8
  Data Type Conversion2 : DataTypeConversion  OutDataTypeStr=uint8
  Dspl : Subsystem
  Gain{1..8} (8 alike) : Gain  Gain=-1  OutDataTypeStr=single
  Ground : Ground
  Ground1 : Ground
  Ground2 : Ground
  Subsystem : Subsystem
  Subsystem1 : Subsystem
  Switch : Switch  Criteria=u2 > Threshold  OutDataTypeStr=uint16
  Switch1 : Switch  Criteria=u2 > Threshold  OutDataTypeStr=uint16
  Switch2 : Switch  Criteria=u2 ~= 0  OutDataTypeStr=uint16
  Switch3 : Switch  Criteria=u2 > Threshold  OutDataTypeStr=uint16
  Switch4 : Switch  Criteria=u2 ~= 0
  Terminator{1..14} (14 alike) : Terminator
  Dspl_stTxtDspl : Outport
  Dspl_stICAIcon : Outport  Port=2
  TSR_Version_Only_Sign_Type : Outport  Port=3
  Vehiclr_Line_Display : Outport  Port=4
  ISA_Value : Outport  Port=5
  Hands_off_warning : Outport  Port=6
  stHWAmode : Outport  Port=7
  LightControlValid : Outport  Port=8
  TurnLightsCmd : Outport  Port=9
  HWAActionSts : Outport  Port=10
  HWATurnOnIndicator : Outport  Port=11
  wires:
  R0C3_Org/1 -> Gain1/1
  L0C0_Org/1 -> Gain7/1
  stTHFKeyStt/1 -> Data Type Conversion16/1
  [L0QI_Opt] -> Terminator6/1
  Dspl/6(Dspl_stVocDspl) -> Hands_off_warning/1
  stLCScene/1 -> Switch1/3
  stTHMode/1 -> Data Type Conversion6/1, Switch/3
  L0QI_Opt/1 -> [L0QI_Opt], Data Type Conversion22/1
  Ground2/1 -> Compare To Zero1/1
  stTHState/1 -> Data Type Conversion35/1
  stSWALimFlg/1 -> Data Type Conversion37/1
  [R0QI_Opt] -> Terminator14/1
  R0C0_Org/1 -> Gain8/1
  L0C2_Org/1 -> Gain5/1
  Ground1/1 -> Data Type Conversion40/1
  VehMovRx_VehicleStationary/1 -> Compare To Zero2/1
  Data Type Conversion24/1 -> Dspl/4(Dspl_facmR0Ql)
  R0QI_Opt/1 -> [R0QI_Opt], Data Type Conversion24/1
  R0C1_Org/1 -> Gain3/1
  Compare To Zero1/1 -> Data Type Conversion36/1
  Data Type Conversion39/1 -> Dspl/6(Dspl_facmL0Type)
  Data Type Conversion37/1 -> Dspl/14(DsplPrcs_stSWALimFlg)
  L0C3_Org/1 -> Gain4/1
  Data Type Conversion17/1 -> Dspl/12(Dspl_tfAddVocCmd)
  Bus Selector1/6 -> Data Type Conversion45/1  "<LCScene_tmp>"
  Data Type Conversion16/1 -> Dspl/10(Dspl_stTHFKeyState)
  EPSRx_stTkOvStChk/1 -> Data Type Conversion38/1
  [bsHMI_Clb] -> Bus Selector1/1
  Data Type Conversion45/1 -> Switch1/1, Switch1/2
  Data Type Conversion36/1 -> Dspl/13(DsplPrcs_dDgrdIconWarnflag)
  HMI_Clb/1 -> [bsHMI_Clb], Dspl/11(DsplPrcs_CIb)
  Data Type Conversion40/1 -> Dspl/7(Dspl_facmR0Type)
  Bus Selector1/2 -> Subsystem/4(Low_Time)  "<TH_HMIClb_tiDgrdIconWarnLoDurT_C>"
  Count1/1(count_out) -> Data Type Conversion/1
  EPSRx_stHandOff/1 -> Data Type Conversion14/1
  Dspl/3(Dspl_stLaneDspl) -> Subsystem/1(Vehicle_Line_Display_Org)
  Switch/1 -> Subsystem/7(THMode)
  Data Type Conversion22/1 -> Dspl/3(Dspl_facmL0Ql)
  Data Type Conversion15/1 -> Dspl/5(Dspl_stVehSty)
  Dspl/5(Dspl_stR0DispType) -> Terminator8/1
  Data Type Conversion35/1 -> Dspl/8(Dspl_stTHState)
  Data Type Conversion14/1 -> Dspl/1(TxHndOff)
  Dspl/4(Dspl_stL0DispType) -> Terminator7/1
  L0C1_Org/1 -> Gain6/1
  Ground/1 -> Data Type Conversion39/1
  Bus Selector1/1 -> Subsystem/3(High_Time)  "<TH_HMIClb_tiDgrdIconWarnHiDurT_C>"
  Gain2/1 -> Terminator12/1
  Gain3/1 -> Terminator11/1
  Gain7/1 -> Terminator2/1
  R0C2_Org/1 -> Gain2/1
  Gain6/1 -> Terminator3/1
  Gain5/1 -> Terminator4/1
  Gain8/1 -> Terminator10/1
  Switch1/1 -> Subsystem/8(LC_Scene)
  Gain1/1 -> Terminator13/1
  HMI_tfAddVocCmd/1 -> Data Type Conversion17/1
  Subsystem/1(TSR_Version_Only_Sign_Type) -> TSR_Version_Only_Sign_Type/1
  Bus Selector1/3 -> Subsystem/5(ISA_Value)  "<ISA_Value>"
  Subsystem/3(ISA Value) -> ISA_Value/1
  Bus Selector1/4 -> Subsystem/6(ISA_Type)  "<ISA_TYPE>"
  Subsystem/2(Vehicle_Line_Display) -> Vehiclr_Line_Display/1
  Data Type Conversion38/1 -> Dspl/2(Dspl_stTkOvStChk)
  Data Type Conversion/1 -> Terminator9/1  "System_Count"
  Gain4/1 -> Terminator5/1
  Bus Selector1/5 -> Switch/1, Switch/2  "<Mode_tmp>"
  Bus Creator/1 -> Dspl/9(Dspl_bsFromFMCMsg)
  Data Type Conversion2/1 -> Bus Creator/2  "ACC_HMI_Txt_Disp"
  Data Type Conversion1/1 -> Bus Creator/1  "ACC_State"
  ACC_HMI_Txt_Disp/1 -> Data Type Conversion2/1
  ACC_State/1 -> Data Type Conversion1/1
  Dspl/1(Dspl_stTxtDspl) -> Dspl_stTxtDspl/1
  Dspl/2(Dspl_stICAIcon) -> Dspl_stICAIcon/1
  Subsystem1/1(TurnLightsCmd) -> HWATurnOnIndicator/1, Switch3/1
  Compare To Zero2/1 -> Data Type Conversion15/1
  stLCmode/1 -> Switch2/1
  stLCfailedFlg/1 -> Terminator1/1
  stLCRmode_valid/1 -> Data Type Conversion3/1
  stturn_lightState/1 -> Data Type Conversion4/1
  stTLC_ALCmodeSW/1 -> Data Type Conversion5/1
  Data Type Conversion4/1 -> Dspl/15(Dspl_stturn_lightState)
  Data Type Conversion5/1 -> Dspl/16(Dspl_stTLC_ALCmodeSW)
  Data Type Conversion6/1 -> Compare To Constant/1
  Compare To Constant/1 -> Switch2/2
  Constant/1 -> Switch2/3
  Switch2/1 -> HWAActionSts/1
  stLC_SpdCndtFlg/1 -> Data Type Conversion7/1
  Data Type Conversion7/1 -> Dspl/17(Dspl_stLC_SpdCndtFlg)
  Dspl/7(Dspl_stHWAmode) -> stHWAmode/1
  Switch3/1 -> TurnLightsCmd/1
  Constant1/1 -> Switch3/3
  stLCRMode/1 -> Subsystem1/1(LCRMode), Subsystem/2(LCRMode)
  Data Type Conversion3/1 -> Switch4/3
  Switch4/1 -> LightControlValid/1, Switch3/2
  Constant2/1 -> Switch4/1
  Constant3/1 -> Switch4/2

== system MIL4L3_SW6_V1_20220211/CarMaker/VehicleControl/OMAP/OMAP1/Runnable_OMAP_10ms_sys/OMAP_Module/ICA_Direct_G59/ICA_Define/TH_HMIClb ==
  note: Level: 3
      | Num: THC.06
      | Rev: 00.00.01
      | Ud: 19-03-28
  Bus Creator1 : BusCreator  Inputs=15
  Constant : Constant  Value=0.01  OutDataTypeStr=single
  Data Type Conversion{,1..7} (8 alike) : DataTypeConversion  OutDataTypeStr=single
  Data Type Conversion{10..13} (4 alike) : DataTypeConversion  OutDataTypeStr=uint16
  ISA_TYPE : Subsystem
      mask Display:
      | port_label('input', 1, 'In');
      | port_label('output', 1, 'Out');
      | color('blue');
      | text(0.5,0.5,'0.789','horizontalAlignment','center');
  ISA_Value : Subsystem
      mask Display:
      | port_label('input', 1, 'In');
      | port_label('output', 1, 'Out');
      | color('blue');
      | text(0.5,0.5,'0.789','horizontalAlignment','center');
  LCScene_tmp : Subsystem
      mask Display:
      | port_label('input', 1, 'In');
      | port_label('output', 1, 'Out');
      | color('blue');
      | text(0.5,0.5,'0.789','horizontalAlignment','center');
  Mode_tmp : Subsystem
      mask Display:
      | port_label('input', 1, 'In');
      | port_label('output', 1, 'Out');
      | color('blue');
      | text(0.5,0.5,'0.789','horizontalAlignment','center');
  TH_HMIClb_tiDgrdIconWarnHiDurT_C : Subsystem
      mask Display:
      | port_label('input', 1, 'In');
      | port_label('output', 1, 'Out');
      | color('blue');
      | text(0.5,0.5,'0.789','horizontalAlignment','center');
  TH_HMIClb_tiDgrdIconWarnLoDurT_C : Subsystem
      mask Display:
      | port_label('input', 1, 'In');
      | port_label('output', 1, 'Out');
      | color('blue');
      | text(0.5,0.5,'0.789','horizontalAlignment','center');
  TH_HMIClb_tiDgrdVocWarnDurT_C : Subsystem
      mask Display:
      | port_label('input', 1, 'In');
      | port_label('output', 1, 'Out');
      | color('blue');
      | text(0.5,0.5,'0.789','horizontalAlignment','center');
  "TH_HMIClb_tiHndOffTxtWarnT_C " : Subsystem
      mask Display:
      | port_label('input', 1, 'In');
      | port_label('output', 1, 'Out');
      | color('blue');
      | text(0.5,0.5,'0.789','horizontalAlignment','center');
  TH_HMIClb_tiHndOffVocWarnT_C : Subsystem
      mask Display:
      | port_label('input', 1, 'In');
      | port_label('output', 1, 'Out');
      | color('blue');
      | text(0.5,0.5,'0.789','horizontalAlignment','center');
  TH_HMIClb_tiSWALimFlgDetT_C : Subsystem
      mask Display:
      | port_label('input', 1, 'In');
      | port_label('output', 1, 'Out');
      | color('blue');
      | text(0.5,0.5,'0.789','horizontalAlignment','center');
  TH_HMIClb_tiTxtLimT_C : Subsystem
      mask Display:
      | port_label('input', 1, 'In');
      | port_label('output', 1, 'Out');
      | color('blue');
      | text(0.5,0.5,'0.789','horizontalAlignment','center');
  Out : Outport
  wires:
  Bus Creator1/1 -> Out/1
  "TH_HMIClb_tiHndOffTxtWarnT_C "/1(Out1) -> Bus Creator1/1  "TH_HMIClb_tiHndOffTxtWarnT_C"
  Data Type Conversion3/1 -> "TH_HMIClb_tiHndOffTxtWarnT_C "/1(In2)
  TH_HMIClb_tiHndOffVocWarnT_C/1(Out1) -> Bus Creator1/2  "TH_HMIClb_tiHndOffVocWarnT_C"
  Data Type Conversion1/1 -> TH_HMIClb_tiHndOffVocWarnT_C/1(In2)
  TH_HMIClb_tiDgrdVocWarnDurT_C/1(Out1) -> Bus Creator1/3  "TH_HMIClb_tiDgrdVocWarnDurT_C"
  Data Type Conversion2/1 -> TH_HMIClb_tiDgrdVocWarnDurT_C/1(In2)
  TH_HMIClb_tiTxtLimT_C/1(Out1) -> Bus Creator1/4  "TH_HMIClb_tiTxtLimT_C"
  Data Type Conversion4/1 -> TH_HMIClb_tiTxtLimT_C/1(In2)
  Data Type Conversion/1 -> Bus Creator1/5  "TH_HMIClb_tiCalcPer_C"
  TH_HMIClb_tiDgrdIconWarnHiDurT_C/1(Out1) -> Bus Creator1/6  "TH_HMIClb_tiDgrdIconWarnHiDurT_C"
  Data Type Conversion5/1 -> TH_HMIClb_tiDgrdIconWarnHiDurT_C/1(In2)
  TH_HMIClb_tiDgrdIconWarnLoDurT_C/1(Out1) -> Bus Creator1/7  "TH_HMIClb_tiDgrdIconWarnLoDurT_C"
  Data Type Conversion6/1 -> TH_HMIClb_tiDgrdIconWarnLoDurT_C/1(In2)
  TH_HMIClb_tiSWALimFlgDetT_C/1(Out1) -> Bus Creator1/8  "TH_HMIClb_tiSWALimFlgDetT_C"
  Data Type Conversion7/1 -> TH_HMIClb_tiSWALimFlgDetT_C/1(In2)
  LCScene_tmp/1(Out1) -> Bus Creator1/11  "LCScene_tmp"
  Data Type Conversion10/1 -> LCScene_tmp/1(In2)  "LCScene_tmp"
  Data Type Conversion12/1 -> ISA_TYPE/1(In2)  "ISA_TYPE"
  ISA_TYPE/1(Out1) -> Bus Creator1/13  "ISA_TYPE"
  ISA_Value/1(Out1) -> Bus Creator1/14  "ISA_Value"
  Data Type Conversion13/1 -> ISA_Value/1(In2)  "ISA_Value"
  Mode_tmp/1(Out1) -> Bus Creator1/15  "Mode_tmp"
  Data Type Conversion11/1 -> Mode_tmp/1(In2)
  Constant/1 -> Data Type Conversion/1

== system MIL4L3_SW6_V1_20220211/CarMaker/VehicleControl/Function/LKA/LKAS1/LL/LL Inputs Mapping/bsLaneInfo/LaneSelect/Subsystem ==
  R0_Q_In : Inport
  Constant1 : Constant  Value=3  OutDataTypeStr=uint8
  Switch1 : Switch  Threshold=2
  R0_Q : Outport
  wires:
  Switch1/1 -> R0_Q/1  "R0_Q"
  R0_Q_In/1 -> Switch1/3, Switch1/2
  Constant1/1 -> Switch1/1

== system MIL4L3_SW6_V1_20220211/CarMaker/VehicleControl/Function/LKA/LKAS1/LL/LL Inputs Mapping/bsLaneInfo/LaneSelect/Subsystem1 ==
  L1_Q_In : Inport
  Constant1 : Constant  Value=3  OutDataTypeStr=uint8
  Switch1 : Switch  Threshold=2
  L1_Q : Outport
  wires:
  Constant1/1 -> Switch1/1
  L1_Q_In/1 -> Switch1/2, Switch1/3
  Switch1/1 -> L1_Q/1  "L1_Q"

== system MIL4L3_SW6_V1_20220211/CarMaker/VehicleControl/Function/LKA/LKAS1/LL/LL Inputs Mapping/bsLaneInfo/LaneSelect/Subsystem2 ==
  R1_Q_In : Inport
  Constant1 : Constant  Value=3  OutDataTypeStr=uint8
  Switch1 : Switch  Threshold=2
  R1_Q : Outport
  wires:
  Switch1/1 -> R1_Q/1  "R1_Q"
  R1_Q_In/1 -> Switch1/3, Switch1/2
  Constant1/1 -> Switch1/1

== system MIL4L3_SW6_V1_20220211/CarMaker/VehicleControl/Function/LKA/LKAS1/LL/LL Inputs Mapping/bsLaneInfo/LaneSelect/Subsystem4 ==
  L0_Q_In : Inport
  Constant : Constant  Value=3  OutDataTypeStr=uint8
  Switch : Switch  Threshold=2
  L0_Q : Outport
  wires:
  Switch/1 -> L0_Q/1  "L0_Q"
  Constant/1 -> Switch/1
  L0_Q_In/1 -> Switch/2, Switch/3

== system MIL4L3_SW6_V1_20220211/CarMaker/VehicleControl/Function/LKA/LKAS1/LL/LL Inputs Mapping/bsLaneInfo/LanesReconstruct /Left 1Lane Reconstruct (Lft1LaneR) ==
  stFlag : Inport
  bsL1Info : Inport  Port=2
  Bus Creator2 : BusCreator  Inputs=8
  Bus Selector1 : BusSelector  OutputSignals=L1_C0,L1_C1,L1_C2,L1_C3,L1_VR,L1_Q,L1_Type,L1_W
  Constant : Constant  Value=0  OutDataTypeStr=uint16
  Switch3 : Switch  Criteria=u2 > Threshold
  bsL1InfoR : Outport
  wires:
  Bus Selector1/8 -> Bus Creator2/8  "<L1_W>"
  Bus Selector1/7 -> Bus Creator2/7  "<L1_Type>"
  Bus Selector1/5 -> Bus Creator2/5  "<L1_VR>"
  bsL1Info/1 -> Bus Selector1/1
  stFlag/1 -> Switch3/2
  Bus Selector1/6 -> Switch3/1  "<L1_Q>"
  Constant/1 -> Switch3/3
  Switch3/1 -> Bus Creator2/6  "L1_Q"
  Bus Creator2/1 -> bsL1InfoR/1  "bsL1Info"
  Bus Selector1/4 -> Bus Creator2/4  "<L1_C3>"
  Bus Selector1/3 -> Bus Creator2/3  "<L1_C2>"
  Bus Selector1/2 -> Bus Creator2/2  "<L1_C1>"
  Bus Selector1/1 -> Bus Creator2/1  "<L1_C0>"

== system MIL4L3_SW6_V1_20220211/CarMaker/VehicleControl/Function/LKA/LKAS1/LL/LL Inputs Mapping/bsLaneInfo/LanesReconstruct /Left Lane Reconstruct (LftLaneR) ==
  lRoadW : Inport
  bsR0Info : Inport  Port=2
  bsL0Info : Inport  Port=3
  Add : Sum  Inputs=+-  OutDataTypeStr=single
  Bus Creator : BusCreator  Inputs=8
  Bus Selector1 : BusSelector  OutputSignals=L0_Q
  Bus Selector3 : BusSelector  OutputSignals=R0_C0,R0_C1,R0_C2,R0_C3,R0_VR,R0_Type,R0_W
  Cast To Single{1..4,6} (5 alike) : DataTypeConversion  OutDataTypeStr=single  LockScale=on
  Cast To Single5 : DataTypeConversion  OutDataTypeStr=uint8  LockScale=on
  Gain : Gain  Gain=-1  OutDataTypeStr=Inherit: Same as input
  bsL0InfoR : Outport
  wires:
  Cast To Single4/1 -> Bus Creator/5  "L0_VR"
  Cast To Single6/1 -> Bus Creator/8  "L0_W"
  Cast To Single5/1 -> Bus Creator/7  "L0_Type"
  Bus Selector3/7 -> Cast To Single6/1  "<R0_W>"
  Bus Selector3/6 -> Cast To Single5/1  "<R0_Type>"
  lRoadW/1 -> Add/1
  bsR0Info/1 -> Bus Selector3/1
  Bus Selector3/1 -> Add/2  "<R0_C0>"
  Add/1 -> Gain/1
  Bus Selector3/2 -> Cast To Single1/1  "<R0_C1>"
  Bus Selector3/3 -> Cast To Single2/1  "<R0_C2>"
  Bus Selector3/4 -> Cast To Single3/1  "<R0_C3>"
  Bus Selector3/5 -> Cast To Single4/1  "<R0_VR>"
  bsL0Info/1 -> Bus Selector1/1
  Bus Selector1/1 -> Bus Creator/6  "<L0_Q>"
  Gain/1 -> Bus Creator/1  "L0_C0"
  Cast To Single1/1 -> Bus Creator/2  "L0_C1"
  Cast To Single2/1 -> Bus Creator/3  "L0_C2"
  Cast To Single3/1 -> Bus Creator/4  "L0_C3"
  Bus Creator/1 -> bsL0InfoR/1  "bsL0Info"

== system MIL4L3_SW6_V1_20220211/CarMaker/VehicleControl/Function/LKA/LKAS1/LL/LL Inputs Mapping/bsLaneInfo/LanesReconstruct /Right 1Lane Reconstruct (Rgt1LaneR) ==
  stFlag : Inport
  bsR1Info : Inport  Port=2
  Bus Creator3 : BusCreator  Inputs=8
  Bus Selector1 : BusSelector  OutputSignals=R1_C0,R1_C1,R1_C2,R1_C3,R1_VR,R1_Q,R1_Type,R1_W
  Constant : Constant  Value=0  OutDataTypeStr=uint16
  Switch3 : Switch  Criteria=u2 > Threshold
  bsL1InfoR : Outport
  wires:
  Bus Selector1/8 -> Bus Creator3/8  "<R1_W>"
  Bus Selector1/7 -> Bus Creator3/7  "<R1_Type>"
  Bus Selector1/5 -> Bus Creator3/5  "<R1_VR>"
  Bus Selector1/1 -> Bus Creator3/1  "<R1_C0>"
  Bus Selector1/2 -> Bus Creator3/2  "<R1_C1>"
  Bus Selector1/3 -> Bus Creator3/3  "<R1_C2>"
  Bus Selector1/4 -> Bus Creator3/4  "<R1_C3>"
  Constant/1 -> Switch3/3
  Bus Selector1/6 -> Switch3/1  "<R1_Q>"
  stFlag/1 -> Switch3/2
  bsR1Info/1 -> Bus Selector1/1
  Bus Creator3/1 -> bsL1InfoR/1  "bsR1Info"
  Switch3/1 -> Bus Creator3/6  "R1_Q"
